simulink model "chlnet"  (Simulink 3.00)
settings: Solver=ode45  StartTime=1  StopTime=length(t)  RelTol=1e-3
values from neighbouring files (symbols this model uses):
  maxdata = max([t' p'])    [chlmin.m]
  mindata = min([t' p'])    [chlmin.m]
libraries: ann x1, simulink3 x1
settings Model: OutputTimes=[0:50:3900]  SaveTime=off  SaveOutput=off  Decimation=35*50  RTWOptions="-aEnforceIntegerDowncast=1 -aFoldNonRolledExpr=1 -aInlineInvariantSignals=1 -aInlineParameters=0 -aLocalBlockOutputs=1 -aRollThreshold=5 -aZeroInternalMemoryAtStartup=1 -aZeroExternalMemoryAtStartup=1 -aInitFltsAndDblsToZero=1 -aGenerateReport=0 -aGenCodeOnly=0 -aRTWVerbose=1 -aIncludeHyperlinkInReport=0 -aLaunchReport=0 -aForceParamTrailComments=0 -aGenerateComments=1 -aIgnoreCustomStorageClasses=1 -aIncHierarchyInIds=0 -aMaxRTWIdLen=31 -aShowEliminatedStatements=0 -aPrefixModelToSubsysFcnNames=1 -aIncDataTypeInIds=0 -aInsertBlockDesc=0 -aSimulinkBlockComments=1 -aInlinedPrmAccess=\"Literals\"  -aSuppressErrorStatus=0 -aModelReferenceCompliant=1 -aSupportNonInlinedSFcns=1 -aSupportContinuousTime=1 -aSupportComplex=1 -aSupportNonFinite=1 -aSupportAbsoluteTime=1 -aTargetFcnLib=\"ansi_tfl_tmw.mat\" -aMultiInstanceERTCode=0 -aLogVarNameModifier=\"rt_\" -aIsPILTarget=0 -aCombineOutputUpdateFcns=0 -aGenerateASAP2=0 -aGenerateSampleERTMain=0 -aGenerateFullHeader=1 -aUtilityFuncGeneration=\"Auto\" -aIncludeFileDelimiter=\"Auto\" -aIncludeMdlTerminateFcn=1 -aPurelyIntegerCode=0 -aERTCustomFileBanners=0 -aRTWCAPIStates=0 -aRTWCAPIParams=0 -aRTWCAPISignals=0 -aMatFileLogging=1 -aGenFloatMathFcnCalls=\"ANSI_C\" -aExtModeMexFile=\"ext_comm\" -aExtModeTransport=0 -aExtModeStaticAllocSize=1000000 -aExtModeTesting=0 -aExtModeStaticAlloc=0 -aExtMode=0  -aInitFltsAndDblsToZero=1 -aInitFltsAndDblsToZero=1 -aInitFltsAndDblsToZero=1"  Creator=Giampy  LastModifiedBy=campa

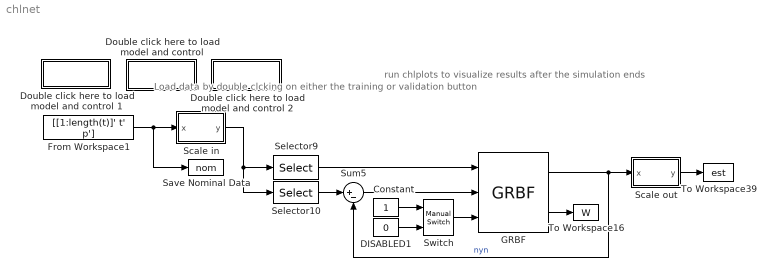
== system chlnet ==
  note: run chlplots to visualize results
      | after the simulation ends
  note: Load data by double clcking on either
      | the training or validation button
  Constant : Constant  Value=1
  DISABLED1 : Constant  Value=0
  "Double click here to load model and control " : Subsystem
      settings: OpenFcn=load choles_all;t=t(:,1:130);p=p(:,1:130);mindata=min([t' p']);maxdata=max([t' p']);W=zeros(1,((21+2)*100+2)*3);
      mask Display: disp('Training\nData')
  Double click here to load model and control 1 : Subsystem
      settings: OpenFcn=edit('training.txt')
      mask Display: disp('Readme')
  Double click here to load model and control 2 : Subsystem
      settings: OpenFcn=load choles_all; t=t(:,131:end);p=p(:,131:end); load chl_W
      mask Display: disp('Validation\nData')
  From Workspace1 : FromWorkspace  VariableName=[[1:length(t)]' t' p']  SampleTime=1  HoldFinalValue=off
  GRBF : ann/GRBF  dim=[21 3]  nwrap="[100   0.4         1e10           1]"  eta=[0.0001 0.0001 0.0001]  gam=[1e-6 1e-6 1e-6]*0  lim=[1e9 1e9 1e9]  e1=0.1  e2="[0.6  0.6  1]"  e3=[0.02 0.5]  x0=W(end,:) % zeros(((21+2)*100+2)*3,1) %  T=1
  Save Nominal Data : ToWorkspace  VariableName=nom  SampleTime=1  SaveFormat=Matrix
      settings: Buffer=1000
  Scale in : Subsystem  mask(Scale){xmin=mindata, xmax=maxdata, ymin=-ones(size(mindata)), ymax=ones(size(maxdata))}
      mask prompts: xmin "x min"; xmax "x max"; ymin "y min"; ymax "y max"
      mask help:
      | Scales the input vector x, ranging from xmin to xmax,
      |    to an output vector y, ranging from ymin to ymax
      mask Help:
      | Scales the input vector x, ranging from xmin to xmax,
      |    to an output vector y, ranging from ymin to ymax
  Scale out : Subsystem  mask(Scale){xmin=-ones(1,3), xmax=ones(1,3), ymin=mindata(1:3), ymax=maxdata(1:3)}
      mask prompts: xmin "x min"; xmax "x max"; ymin "y min"; ymax "y max"
      mask help:
      | Scales the input vector x, ranging from xmin to xmax,
      |    to an output vector y, ranging from ymin to ymax
      mask Help:
      | Scales the input vector x, ranging from xmin to xmax,
      |    to an output vector y, ranging from ymin to ymax
  Selector10 : Selector  Elements=1:3  InputPortWidth=24
  Selector9 : Selector  Elements=4:24  InputPortWidth=24
  Sum5 : Sum  Inputs=|+-  SaturateOnIntegerOverflow=on
  Switch : simulink3/Nonlinear/Manual Switch  sw=1  action=0
  To Workspace16 : ToWorkspace  VariableName=W  SampleTime=1  SaveFormat=Matrix
      settings: Buffer=1000
  To Workspace39 : ToWorkspace  VariableName=est  SampleTime=1  SaveFormat=Matrix
      settings: Buffer=1000
  wires:
  From Workspace1/1 -> Save Nominal Data/1, Scale in/1(x)
  Scale in/1(y) -> Selector9/1, Selector10/1
  Selector10/1 -> Sum5/1
  Selector9/1 -> GRBF/1
  Scale out/1(y) -> To Workspace39/1
  GRBF/1 -> Sum5/2, Scale out/1(x)  "nyn"
  GRBF/2 -> To Workspace16/1
  Constant/1 -> Switch/1
  DISABLED1/1 -> Switch/2
  Sum5/1 -> GRBF/2
  Switch/1 -> GRBF/3

== system chlnet/Double click here to load model and control  ==

== system chlnet/Double click here to load model and control 1 ==

== system chlnet/Double click here to load model and control 2 ==

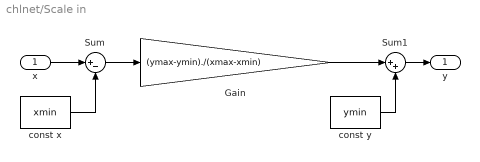
== system chlnet/Scale in ==
  x : Inport  Port=1  PortWidth=-1  SampleTime=-1  DataType=auto
      settings: SignalType=auto
  Gain : Gain  Gain=(ymax-ymin)./(xmax-xmin)  SaturateOnIntegerOverflow=on
  Sum : Sum  Inputs=|+-  SaturateOnIntegerOverflow=on
  Sum1 : Sum  Inputs=|++  SaturateOnIntegerOverflow=on
  const x : Constant  Value=xmin
  const y : Constant  Value=ymin
  y : Outport  Port=1
  wires:
  x/1 -> Sum/1
  Sum/1 -> Gain/1
  const x/1 -> Sum/2
  Gain/1 -> Sum1/1
  Sum1/1 -> y/1
  const y/1 -> Sum1/2

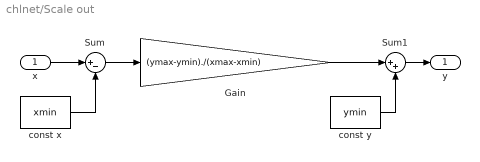
== system chlnet/Scale out ==
  x : Inport  Port=1  PortWidth=-1  SampleTime=-1  DataType=auto
      settings: SignalType=auto
  Gain : Gain  Gain=(ymax-ymin)./(xmax-xmin)  SaturateOnIntegerOverflow=on
  Sum : Sum  Inputs=|+-  SaturateOnIntegerOverflow=on
  Sum1 : Sum  Inputs=|++  SaturateOnIntegerOverflow=on
  const x : Constant  Value=xmin
  const y : Constant  Value=ymin
  y : Outport  Port=1
  wires:
  const y/1 -> Sum1/2
  Sum1/1 -> y/1
  Gain/1 -> Sum1/1
  const x/1 -> Sum/2
  Sum/1 -> Gain/1
  x/1 -> Sum/1
